simulink model "CAVE_MachE_Testing_testing_V2"  (R2024a)
settings: configuration reference "ConfigSetDesktopFixedStep" (kept outside this file)
PreLoadFcn:
  | VSS_BICYCLE=Simulink.Variant('Dual=0');
  | VSS_DUAL=Simulink.Variant('Dual=1');
  | Dual=1;
  | load('DriveCycle2.mat')
PostLoadFcn:
  | if any(exist('dsrtsu_mdlpostloadfcn', 'file') ~= 0), dsrtsu_mdlpostloadfcn('Execute', bdroot); end
InitFcn:
  | , if any(exist('rtifpga_mdlclblib', 'file') ~= 0), rtifpga_mdlclblib('Init', bdroot); end,
  | , if any(exist('dsmpb_private', 'file') ~= 0), dsmpb_private('dsmpb_mdlclblib', 'Init', bdroot); end,
  | load('DriveCycle2.mat')
model workspace (MAT data in the model file):
  Gas = 0.383333333333
undefined symbols (not defined in the file or in its folder): AccelCmd, ActTqLF_Nm_, ActTqLR_Nm_, ActTqRF_Nm_, ActTqRR_Nm_, BattChargeLimitMaxPwr, BattChargeLimitSocBpts, BattChargeLimitTbl, BattChrgCapcty, BattDischargeLimitSocBpts, BattDischargeLimitTbl, BattDischargeMaxPwr, BattNumCellsParallel, BattNumCellsSeries, BattOpenVoltCapBpts, BattOpenVoltTbl, BattResistSocBpts, BattResistTbl, BattResistTempBpts, BrakeMaxPrs, BrakeMaxTrq, ChassisDistCg2FrontAxle, ChassisDistCg2RearAxle, ChassisVehMass, CltchCmd, CoastDown, DecelCmd, DiffRatio, DiscIntNeverNeededParam, EnvGravCnst, EnvPrs, EnvTemp, FuelSpecificGrav, GearCmd, h, InitStates, lgSw, limitedMCT, MCT, MtrEffSpdBpts, MtrEffTbl, MtrEffTrqBpts, MtrPwrMax, MtrTrqMax, out_1, pMCT, RealSimPara, Ref_speed, Ref_time, SteeringCmd, SupvsryCtrlRegenBrkCutOffTbl, SupvsryCtrlRegenSpdBpts, TestScnrioCycleNum, US06, VEH
libraries: VSIGenLib x65, simulink x54, etargetslib x38, dsmpblib x24, vehdynlibtire x12, autolibshared x11, vehdynlibsuspension x7, vehdynlibtirecommon x7, autolibpowerinfoutils x6, autolibutils x5, autolibsharedcoupling x4, autolibmappedmotor x4
(part 9 of 17)

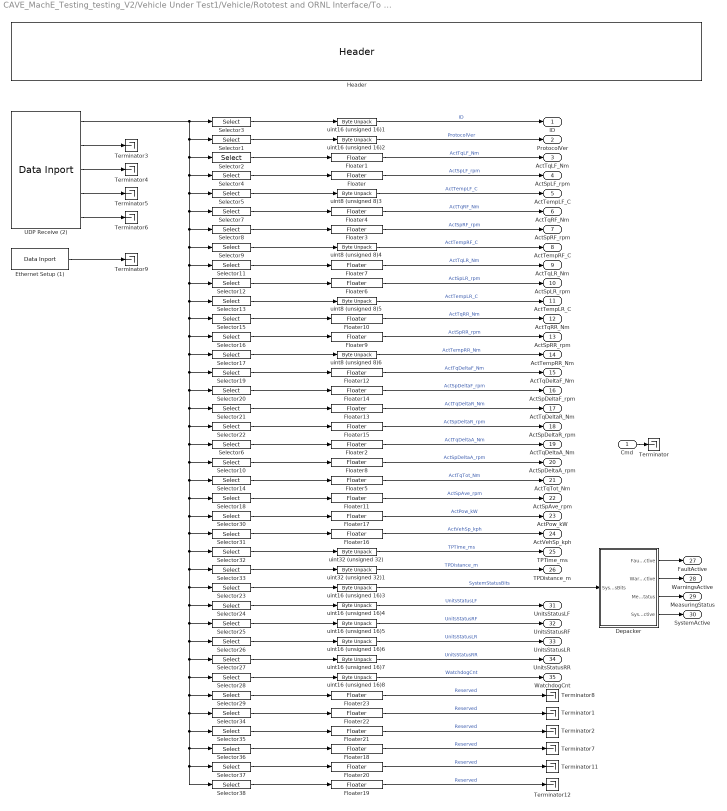
== system CAVE_MachE_Testing_testing_V2/Vehicle Under Test1/Vehicle/Rototest and ORNL Interface/To Rototest with Band-Aid/Logging/RotoTestEthRXLogging ==
  Cmd : Inport
  Depacker : Subsystem
  Ethernet Setup (1) : dsmpblib/Data Inport  Priority=10000
      settings: SourceProductName=dSPACE Model Interface Package for Simulink (MIPS)
  Floater{,1..23} (24 alike) : VSIGenLib/Floater  SystemSampleTime=-1  VariantActivationTime=update diagram  AllowFlexibleInterface=on  Latency=0  AutoFrameSizeCalculation=off
  Header : VSIGenLib/Header  not=''
  Selector1 : Selector  IndexMode=Zero-based  InputPortWidth=124  IndexOptions=Index vector (dialog)  Indices=[3 2]  OutputSizes=1
  Selector10 : Selector  IndexMode=Zero-based  InputPortWidth=124  IndexOptions=Index vector (dialog)  Indices=[63 62 61 60]  OutputSizes=1
  Selector11 : Selector  IndexMode=Zero-based  InputPortWidth=124  IndexOptions=Index vector (dialog)  Indices=[25 24 23 22]  OutputSizes=1
  Selector12 : Selector  IndexMode=Zero-based  InputPortWidth=124  IndexOptions=Index vector (dialog)  Indices=[29 28 27 26]  OutputSizes=1
  Selector13 : Selector  IndexMode=Zero-based  InputPortWidth=124  IndexOptions=Index vector (dialog)  Indices=[30]  OutputSizes=1
  Selector14 : Selector  IndexMode=Zero-based  InputPortWidth=124  IndexOptions=Index vector (dialog)  Indices=[67 66 65 64]  OutputSizes=1
  Selector15 : Selector  IndexMode=Zero-based  InputPortWidth=124  IndexOptions=Index vector (dialog)  Indices=[34 33 32 31]  OutputSizes=1
  Selector16 : Selector  IndexMode=Zero-based  InputPortWidth=124  IndexOptions=Index vector (dialog)  Indices=[38 37 36 35]  OutputSizes=1
  Selector17 : Selector  IndexMode=Zero-based  InputPortWidth=124  IndexOptions=Index vector (dialog)  Indices=[39]  OutputSizes=1
  Selector18 : Selector  IndexMode=Zero-based  InputPortWidth=124  IndexOptions=Index vector (dialog)  Indices=[71 70 69 68]  OutputSizes=1
  Selector19 : Selector  IndexMode=Zero-based  InputPortWidth=124  IndexOptions=Index vector (dialog)  Indices=[43 42 41 40]  OutputSizes=1
  Selector2 : Selector  IndexMode=Zero-based  InputPortWidth=124  IndexOptions=Index vector (dialog)  Indices=[7 6 5 4]  OutputSizes=1
  Selector20 : Selector  IndexMode=Zero-based  InputPortWidth=124  IndexOptions=Index vector (dialog)  Indices=[47 46 45 44]  OutputSizes=1
  Selector21 : Selector  IndexMode=Zero-based  InputPortWidth=124  IndexOptions=Index vector (dialog)  Indices=[51 50 49 48]  OutputSizes=1
  Selector22 : Selector  IndexMode=Zero-based  InputPortWidth=124  IndexOptions=Index vector (dialog)  Indices=[55 54 53 52]  OutputSizes=1
  Selector23 : Selector  IndexMode=Zero-based  InputPortWidth=124  IndexOptions=Index vector (dialog)  Indices=[89 88]  OutputSizes=1
  Selector24 : Selector  IndexMode=Zero-based  InputPortWidth=124  IndexOptions=Index vector (dialog)  Indices=[91 90]  OutputSizes=1
  Selector25 : Selector  IndexMode=Zero-based  InputPortWidth=124  IndexOptions=Index vector (dialog)  Indices=[93 92]  OutputSizes=1
  Selector26 : Selector  IndexMode=Zero-based  InputPortWidth=124  IndexOptions=Index vector (dialog)  Indices=[95 94]  OutputSizes=1
  Selector27 : Selector  IndexMode=Zero-based  InputPortWidth=124  IndexOptions=Index vector (dialog)  Indices=[97 96]  OutputSizes=1
  Selector28 : Selector  IndexMode=Zero-based  InputPortWidth=124  IndexOptions=Index vector (dialog)  Indices=[99 98]  OutputSizes=1
  Selector29 : Selector  IndexMode=Zero-based  InputPortWidth=124  IndexOptions=Index vector (dialog)  Indices=[103 102 101 100]  OutputSizes=1
  Selector3 : Selector  IndexMode=Zero-based  InputPortWidth=124  IndexOptions=Index vector (dialog)  Indices=[1 0]  OutputSizes=1
  Selector30 : Selector  IndexMode=Zero-based  InputPortWidth=124  IndexOptions=Index vector (dialog)  Indices=[67 66 65 64]  OutputSizes=1
  Selector31 : Selector  IndexMode=Zero-based  InputPortWidth=124  IndexOptions=Index vector (dialog)  Indices=[71 70 69 68]  OutputSizes=1
  Selector32 : Selector  IndexMode=Zero-based  InputPortWidth=124  IndexOptions=Index vector (dialog)  Indices=[83 82 81 80]  OutputSizes=1
  Selector33 : Selector  IndexMode=Zero-based  InputPortWidth=124  IndexOptions=Index vector (dialog)  Indices=[87 86 85 84]  OutputSizes=1
  Selector34 : Selector  IndexMode=Zero-based  InputPortWidth=124  IndexOptions=Index vector (dialog)  Indices=[107 106 105 104]  OutputSizes=1
  Selector35 : Selector  IndexMode=Zero-based  InputPortWidth=124  IndexOptions=Index vector (dialog)  Indices=[111 110 109 108]  OutputSizes=1
  Selector36 : Selector  IndexMode=Zero-based  InputPortWidth=124  IndexOptions=Index vector (dialog)  Indices=[115 114 113 112]  OutputSizes=1
  Selector37 : Selector  IndexMode=Zero-based  InputPortWidth=124  IndexOptions=Index vector (dialog)  Indices=[119 118 117 116]  OutputSizes=1
  Selector38 : Selector  IndexMode=Zero-based  InputPortWidth=124  IndexOptions=Index vector (dialog)  Indices=[123 122 121 120]  OutputSizes=1
  Selector4 : Selector  IndexMode=Zero-based  InputPortWidth=124  IndexOptions=Index vector (dialog)  Indices=[11 10 9 8]  OutputSizes=1
  Selector5 : Selector  IndexMode=Zero-based  InputPortWidth=124  IndexOptions=Index vector (dialog)  Indices=[12]  OutputSizes=1
  Selector6 : Selector  IndexMode=Zero-based  InputPortWidth=124  IndexOptions=Index vector (dialog)  Indices=[59 58 57 56]  OutputSizes=1
  Selector7 : Selector  IndexMode=Zero-based  InputPortWidth=124  IndexOptions=Index vector (dialog)  Indices=[16 15 14 13]  OutputSizes=1
  Selector8 : Selector  IndexMode=Zero-based  InputPortWidth=124  IndexOptions=Index vector (dialog)  Indices=[20 19 18 17]  OutputSizes=1
  Selector9 : Selector  IndexMode=Zero-based  InputPortWidth=124  IndexOptions=Index vector (dialog)  Indices=[21]  OutputSizes=1
  Terminator{,1..9,11..12} (12 alike) : Terminator
  UDP Receive (2) : dsmpblib/Data Inport  Priority=10000
      settings: SourceProductName=dSPACE Model Interface Package for Simulink (MIPS)
  uint16 (unsigned 16){1..8} (8 alike) : etargetslib/Byte Unpack  dimensions={[1]}  datatypes={'uint16'}  byteAlign=1
  uint32 (unsigned 32) : etargetslib/Byte Unpack  dimensions={[1]}  datatypes={'uint32'}  byteAlign=1
  uint32 (unsigned 32)1 : etargetslib/Byte Unpack  dimensions={[1]}  datatypes={'uint32'}  byteAlign=1
  uint8 (unsigned 8){3..6} (4 alike) : etargetslib/Byte Unpack  dimensions={[1]}  datatypes={'uint8'}  byteAlign=1
  ID : Outport
  ProtocolVer : Outport  Port=2
  ActTqLF_Nm : Outport  Port=3
  ActSpLF_rpm : Outport  Port=4
  ActTempLF_C : Outport  Port=5
  ActTqRF_Nm : Outport  Port=6
  ActSpRF_rpm : Outport  Port=7
  ActTempRF_C : Outport  Port=8
  ActTqLR_Nm : Outport  Port=9
  ActSpLR_rpm : Outport  Port=10
  ActTempLR_C : Outport  Port=11
  ActTqRR_Nm : Outport  Port=12
  ActSpRR_rpm : Outport  Port=13
  ActTempRR_Nm : Outport  Port=14
  ActTqDeltaF_Nm : Outport  Port=15
  ActSpDeltaF_rpm : Outport  Port=16
  ActTqDeltaR_Nm : Outport  Port=17
  ActSpDeltaR_rpm : Outport  Port=18
  ActTqDeltaA_Nm : Outport  Port=19
  ActSpDeltaA_rpm : Outport  Port=20
  ActTqTot_Nm : Outport  Port=21
  ActSpAve_rpm : Outport  Port=22
  ActPow_kW : Outport  Port=23
  ActVehSp_kph : Outport  Port=24
  TPTime_ms : Outport  Port=25
  TPDistance_m : Outport  Port=26
  FaultActive : Outport  Port=27
  WarningsActive : Outport  Port=28
  MeasuringStatus : Outport  Port=29
  SystemActive : Outport  Port=30
  UnitsStatusLF : Outport  Port=31
  UnitsStatusRF : Outport  Port=32
  UnitsStatusLR : Outport  Port=33
  UnitsStatusRR : Outport  Port=34
  WatchdogCnt : Outport  Port=35
  wires:
  Cmd/1 -> Terminator/1
  Floater23/1 -> Terminator8/1  "Reserved"
  Floater22/1 -> Terminator1/1  "Reserved"
  Floater21/1 -> Terminator2/1  "Reserved"
  Floater20/1 -> Terminator11/1  "Reserved"
  Floater19/1 -> Terminator12/1  "Reserved"
  Floater18/1 -> Terminator7/1  "Reserved"
  Selector38/1 -> Floater19/1
  UDP Receive (2)/1 -> Selector7/1, Selector8/1, Selector9/1, Selector11/1, Selector12/1, Selector13/1, Selector15/1, Selector16/1, Selector17/1, Selector19/1, Selector20/1, Selector21/1, Selector22/1, Selector6/1, Selector10/1, Selector14/1, Selector18/1, Selector30/1, Selector31/1, Selector32/1, Selector33/1, Selector23/1, Selector25/1, Selector26/1, Selector27/1, Selector29/1, Selector34/1, Selector35/1, Selector36/1, Selector37/1, Selector38/1, Selector28/1, Selector24/1, Selector5/1, Selector4/1, Selector2/1, Selector1/1, Selector3/1
  Selector37/1 -> Floater20/1
  Selector36/1 -> Floater18/1
  Selector35/1 -> Floater21/1
  Selector34/1 -> Floater22/1
  Selector32/1 -> uint32 (unsigned 32)/1
  Selector33/1 -> uint32 (unsigned 32)1/1
  uint32 (unsigned 32)1/1 -> TPDistance_m/1  "TPDistance_m"
  uint32 (unsigned 32)/1 -> TPTime_ms/1  "TPTime_ms"
  Floater16/1 -> ActVehSp_kph/1  "ActVehSp_kph"
  Selector31/1 -> Floater16/1
  Floater17/1 -> ActPow_kW/1  "ActPow_kW"
  Selector30/1 -> Floater17/1
  Selector6/1 -> Floater2/1
  Selector14/1 -> Floater5/1
  Selector10/1 -> Floater8/1
  Floater5/1 -> ActTqTot_Nm/1  "ActTqTot_Nm"
  Selector18/1 -> Floater11/1
  Floater2/1 -> ActTqDeltaA_Nm/1  "ActTqDeltaA_Nm"
  Floater8/1 -> ActSpDeltaA_rpm/1  "ActSpDeltaA_rpm"
  Floater11/1 -> ActSpAve_rpm/1  "ActSpAve_rpm"
  Ethernet Setup (1)/1 -> Terminator9/1
  Depacker/4(SystemActive) -> SystemActive/1
  Depacker/1(FaultActive) -> FaultActive/1
  Depacker/2(WarningsActive) -> WarningsActive/1
  Depacker/3(MeasuringStatus) -> MeasuringStatus/1
  uint8 (unsigned 8)4/1 -> ActTempRF_C/1  "ActTempRF_C"
  Floater/1 -> ActSpLF_rpm/1  "ActSpLF_rpm"
  uint16 (unsigned 16)1/1 -> ID/1  "ID"
  Floater15/1 -> ActSpDeltaR_rpm/1  "ActSpDeltaR_rpm"
  uint16 (unsigned 16)8/1 -> WatchdogCnt/1  "WatchdogCnt"
  Floater14/1 -> ActSpDeltaF_rpm/1  "ActSpDeltaF_rpm"
  uint16 (unsigned 16)5/1 -> UnitsStatusRF/1  "UnitsStatusRF"
  Floater9/1 -> ActSpRR_rpm/1  "ActSpRR_rpm"
  Floater1/1 -> ActTqLF_Nm/1  "ActTqLF_Nm"
  uint8 (unsigned 8)3/1 -> ActTempLF_C/1  "ActTempLF_C"
  Floater12/1 -> ActTqDeltaF_Nm/1  "ActTqDeltaF_Nm"
  Floater7/1 -> ActTqLR_Nm/1  "ActTqLR_Nm"
  uint16 (unsigned 16)2/1 -> ProtocolVer/1  "ProtocolVer"
  Selector24/1 -> uint16 (unsigned 16)4/1
  Selector7/1 -> Floater4/1
  Selector8/1 -> Floater3/1
  uint16 (unsigned 16)7/1 -> UnitsStatusRR/1  "UnitsStatusRR"
  Selector22/1 -> Floater15/1
  Selector12/1 -> Floater6/1
  Selector23/1 -> uint16 (unsigned 16)3/1
  uint16 (unsigned 16)6/1 -> UnitsStatusLR/1  "UnitsStatusLR"
  Selector17/1 -> uint8 (unsigned 8)6/1
  UDP Receive (2)/3 -> Terminator4/1
  uint16 (unsigned 16)4/1 -> UnitsStatusLF/1  "UnitsStatusLF"
  Selector27/1 -> uint16 (unsigned 16)7/1
  Floater13/1 -> ActTqDeltaR_Nm/1  "ActTqDeltaR_Nm"
  Selector2/1 -> Floater1/1
  Selector13/1 -> uint8 (unsigned 8)5/1
  Selector26/1 -> uint16 (unsigned 16)6/1
  uint16 (unsigned 16)3/1 -> Depacker/1(SysStsBits)  "SystemStatusBits"
  Floater3/1 -> ActSpRF_rpm/1  "ActSpRF_rpm"
  UDP Receive (2)/2 -> Terminator3/1
  Selector25/1 -> uint16 (unsigned 16)5/1
  Floater4/1 -> ActTqRF_Nm/1  "ActTqRF_Nm"
  Selector29/1 -> Floater23/1
  uint8 (unsigned 8)6/1 -> ActTempRR_Nm/1  "ActTempRR_Nm"
  Floater6/1 -> ActSpLR_rpm/1  "ActSpLR_rpm"
  Selector20/1 -> Floater14/1
  Selector9/1 -> uint8 (unsigned 8)4/1
  Selector5/1 -> uint8 (unsigned 8)3/1
  Selector15/1 -> Floater10/1
  Selector16/1 -> Floater9/1
  uint8 (unsigned 8)5/1 -> ActTempLR_C/1  "ActTempLR_C"
  Selector3/1 -> uint16 (unsigned 16)1/1
  UDP Receive (2)/4 -> Terminator5/1
  Selector28/1 -> uint16 (unsigned 16)8/1
  Selector21/1 -> Floater13/1
  Selector19/1 -> Floater12/1
  Selector1/1 -> uint16 (unsigned 16)2/1
  UDP Receive (2)/5 -> Terminator6/1
  Selector4/1 -> Floater/1
  Floater10/1 -> ActTqRR_Nm/1  "ActTqRR_Nm"
  Selector11/1 -> Floater7/1

== system CAVE_MachE_Testing_testing_V2/Vehicle Under Test1/Vehicle/Rototest and ORNL Interface/To Rototest with Band-Aid/RotoTestEthTx/Packer ==
  SpTqRR : Inport
  SpTqLR : Inport  Port=2
  SpTqRF : Inport  Port=3
  SpTqLF : Inport  Port=4
  SystemActive : Inport  Port=5
  Add : Sum  Inputs=++++++++  OutDataTypeStr=uint8
  Bit0 : Gain  OutDataTypeStr=uint8
  Bit1 : Gain  Gain=2  OutDataTypeStr=uint8
  Bit2 : Gain  Gain=4  OutDataTypeStr=Inherit: Inherit via back propagation
  Bit3 : Gain  Gain=8  OutDataTypeStr=uint8
  Bit4 : Gain  Gain=16  OutDataTypeStr=uint8
  Bit5 : Gain  Gain=32  OutDataTypeStr=uint8
  Bit6 : Gain  Gain=64  OutDataTypeStr=uint8
  Bit7 : Gain  Gain=128  OutDataTypeStr=uint8
  Ground11 : Ground
  Header : VSIGenLib/Header  not=''
  SystemCtrlBits : Outport
  wires:
  SpTqRF/1 -> Bit2/1
  SpTqLF/1 -> Bit1/1
  SpTqRR/1 -> Bit4/1
  SpTqLR/1 -> Bit3/1
  Add/1 -> SystemCtrlBits/1  "SystemCtrlBits"
  Bit0/1 -> Add/8  "SystemActive"
  Bit1/1 -> Add/7  "SpTqLF"
  Bit7/1 -> Add/1  "Reserved"
  SystemActive/1 -> Bit0/1
  Bit4/1 -> Add/4  "SpTqRR"
  Bit6/1 -> Add/2  "Reserved"
  Bit3/1 -> Add/5  "SpTqLR"
  Ground11/1 -> Bit7/1, Bit5/1, Bit6/1  "Reserved"
  Bit5/1 -> Add/3  "Reserved"
  Bit2/1 -> Add/6  "SpTqRF"

== system CAVE_MachE_Testing_testing_V2/Vehicle Under Test1/Vehicle/Vehicle Dynamics/Vehicle 14DOF/Subsystem1/Subsystem ==
  Cgxyzdot : Inport
  angles : Inport  Port=2
  Demux2 : Demux  Outputs=3
  Demux3 : Demux  Outputs=3
  Scope : Scope
  Terminator{,1..4} (5 alike) : Terminator
  VehSpd : Outport
  wires:
  Cgxyzdot/1 -> Demux2/1
  Demux3/2 -> Terminator3/1  "theta"
  Demux2/2 -> Scope/1, Terminator/1  "xdot"
  Demux3/1 -> Terminator2/1  "phi"
  Demux3/3 -> Terminator4/1  "psi"
  Demux2/3 -> Terminator1/1  "zdot"
  angles/1 -> Demux3/1
  Demux2/1 -> VehSpd/1  "xdot"

== system CAVE_MachE_Testing_testing_V2/Vehicle Under Test1/Vehicle/Vehicle Dynamics/Vehicle 14DOF/Subsystem4/Subsystem ==
  Cgxyzdot : Inport
  angles : Inport  Port=2
  Demux2 : Demux  Outputs=3
  Demux3 : Demux  Outputs=3
  Terminator{,1..4} (5 alike) : Terminator
  VehSpd : Outport
  wires:
  Demux2/1 -> VehSpd/1  "xdot"
  angles/1 -> Demux3/1
  Demux2/3 -> Terminator1/1  "zdot"
  Demux3/3 -> Terminator4/1  "psi"
  Demux3/1 -> Terminator2/1  "phi"
  Demux2/2 -> Terminator/1  "xdot"
  Demux3/2 -> Terminator3/1  "theta"
  Cgxyzdot/1 -> Demux2/1

== system CAVE_MachE_Testing_testing_V2/Vehicle Under Test1/Vehicle/Vehicle Dynamics/Vehicle 14DOF/Suspension/Double Wishbone Suspension ==
  Wheel : Inport
  Steering : Inport  Port=2
  Vehicle : Inport  Port=3
  Bus Creator1 : BusCreator  Inputs=5
  Bus Creator2 : BusCreator  Inputs=2
  Bus Creator3 : BusCreator  Inputs=2
  Bus Creator4 : BusCreator  Inputs=6
  Bus Selector : BusSelector  OutputSignals=z,Re,zdot,Fx,Fy,M
  Bus Selector1 : BusSelector  OutputSignals=P,V
  Independent Suspension – Double Wishbone : vehdynlibsuspension/Independent Suspension - Double Wishbone  ActiveDampEn=off  NumAxl=2  NumWhlsByAxl=[2 2]  StrgEnByAxl=[1 0]  AntiSwayEnByAxl=[1 0]  WhlNumVec="[1  2  1  2]"  AxleNumVec="[1  1  2  2]"  SuspTypesByAxle="[1  1]"  SuspImage=suspdw.png  IdealSuspEn=on  IdealSuspAxles="[1  2]"  Kz=Kz  F0z=F0z  Cz=Cz  Hmax=Hmax  f_act_susp_cz=[10000 10000;10000 10000]  f_act_susp_duty_bpt=[0 1]  f_act_susp_zdot_bpt=[-1 1]  Toe=0.  RollStrgSlp=0.  ToeStrgSlp=0.  Caster=0.  CasterHslp=0.  CasterStrgSlp=0.  Camber=0.  CamberHslp=0.  CamberStrgSlp=0.  StrgHgtSlp=0.1432  MappedSuspEn=off  MappedSuspAxles="[1  2]"  f_susp_axl_bp=[1 2]  f_susp_dz_bp=[-0.15 -0.14 -0.13 -0.12 -0.11 -0.10 -0.09 -0.08 -0.07 -0.06 -0.05 -0.04 -0.03 -0.02 -0.01 0.00 0.01 0.02 0.03 0.04 0.05 0.06 0.07 0.08 0.09 0.10 0.11 0.12 0.13 0.14 0.15]  f_susp_dzdot_bp=[-0.15 -0.14 -0.13 -0.12 -0.11 -0.10 -0.09 -0.08 -0.07 -0.06 -0.05 -0.04 -0.03 -0.02 -0.01 0.00 0.01 0.02 0.03 0.04 0.05 0.06 0.07 0.08 0.09 0.10 0.11 0.12 0.13 0.14 0.15]  f_susp_fmz=zeros(31,31,61,2,4)  f_susp_geom=zeros(31,61,2,3)  f_susp_strgdelta_bp=[-30,-29,-28,-27,-26,-25,-24,-23,-22,-21,-20,-19,-18,-17,-16,-15,-14,-13,-12,-11,-10,-9,-8,-7,-6,-5,-4,-3,-2,-1,0,1,2,3,4,5,6,7,8,9,10,11,12,13,14,15,16,17,18,19,20,21,22,23,24,25,26,27,28,29,30]  AntiSwayR=0.2  AntiSwayNtrlAng=0.5236  AntiSwayTrsK=8e2
  Selector1 : Selector  NumberOfDimensions=2  IndexOptions=Index vector (dialog),Select all  Indices=1,1  OutputSizes=1,1
  Selector2 : Selector  NumberOfDimensions=2  IndexOptions=Index vector (dialog),Select all  Indices=2,1  OutputSizes=1,1
  Steer Rate Adapter : Subsystem
  Steering Adapter : Subsystem
  Terminator : Terminator
  Vehicle Adapter : Subsystem
  Wheel  Adapter : Subsystem
  Suspension : Outport  VectorParamsAs1DForOutWhenUnconnected=off
  wires:
  Bus Selector/3 -> Independent Suspension – Double Wishbone/3  "<zdot>"
  Wheel  Adapter/1(WhlFx) -> Bus Creator4/1  "Fx"
  Bus Creator1/1 -> Bus Creator3/2  "Whl"
  Independent Suspension – Double Wishbone/6 -> Bus Creator1/4  "Ang"
  Wheel  Adapter/3(z) -> Bus Creator4/3
  Bus Selector/1 -> Independent Suspension – Double Wishbone/1  "<z>"
  Bus Selector/5 -> Independent Suspension – Double Wishbone/5  "<Fy>"
  Bus Selector/6 -> Independent Suspension – Double Wishbone/6  "<M>"
  Vehicle/1 -> Vehicle Adapter/1(Veh), Steer Rate Adapter/1(Veh)
  Wheel  Adapter/4(zdot) -> Bus Creator4/4
  Vehicle Adapter/1(VehSusp) -> Bus Selector1/1
  Independent Suspension – Double Wishbone/3 -> Bus Creator2/2  "M"
  Selector1/1 -> Bus Creator1/2  "xdot"
  Steering/1 -> Steering Adapter/1(Steer)
  Independent Suspension – Double Wishbone/4 -> Bus Creator1/1  "F"
  Bus Selector/4 -> Independent Suspension – Double Wishbone/4  "<Fx>"
  Wheel  Adapter/5(M) -> Bus Creator4/5  "M"
  Bus Selector/2 -> Independent Suspension – Double Wishbone/2  "<Re>"
  Independent Suspension – Double Wishbone/2 -> Bus Creator2/1  "F"
  Bus Selector1/2 -> Independent Suspension – Double Wishbone/8  "<V>"
  Selector2/1 -> Bus Creator1/3  "ydot"
  Independent Suspension – Double Wishbone/5 -> Selector1/1, Selector2/1  "V"
  Bus Creator2/1 -> Bus Creator3/1  "Veh"
  Bus Creator4/1 -> Bus Selector/1
  Steer Rate Adapter/1(AngVel) -> Bus Creator1/5  "AngVel"
  Wheel/1 -> Wheel  Adapter/1(Wheels)
  Wheel  Adapter/2(WhlFy) -> Bus Creator4/2  "Fy"
  Bus Selector1/1 -> Independent Suspension – Double Wishbone/7  "<P>"
  Wheel  Adapter/6(Re) -> Bus Creator4/6
  Independent Suspension – Double Wishbone/1 -> Terminator/1  "Susp"
  Steering Adapter/1(StrgAng) -> Independent Suspension – Double Wishbone/9
  Bus Creator3/1 -> Suspension/1

== system CAVE_MachE_Testing_testing_V2/Vehicle Under Test1/Vehicle/Vehicle Dynamics/Vehicle 14DOF/Suspension/Independent Mapped Front Suspension Mapped Solid Axle Rear Suspension ==
  Wheel : Inport
  Steering : Inport  Port=2
  Vehicle : Inport  Port=3
  Bus Creator1 : BusCreator  Inputs=5
  Bus Creator2 : BusCreator  Inputs=2
  Bus Creator3 : BusCreator  Inputs=2
  Bus Creator4 : BusCreator  Inputs=6
  Bus Selector : BusSelector  OutputSignals=z,Re,zdot,Fx,Fy,M
  Bus Selector1 : BusSelector  OutputSignals=P,V
  Independent Suspension - Mapped : vehdynlibsuspension/Independent Suspension - Mapped  NumAxl=1  NumWhlsByAxl=[2 2]  StrgEnByAxl=1  AntiSwayEnByAxl=1  WhlNumVec="[1  2  1  2]"  AxleNumVec="[1  1]"  SuspTypesByAxle=[2]  SuspImage=suspindmap.png  IdealSuspEn=off  IdealSuspAxles="[1  2]"  Kz=64370  F0z=9810  Cz=10000  Hmax=0.5  Toe=2  RollStrgSlp=-13  ToeStrgSlp=0.01  Caster=4  CasterHslp=-13  CasterStrgSlp=0.01  Camber=4  CamberHslp=-13  CamberStrgSlp=0.01  StrgHgtSlp=0.0025  MappedSuspEn=on  MappedSuspAxles=[1]  f_susp_axl_bp=[1 2]  f_susp_dz_bp=f_susp_dz_bp  f_susp_dzdot_bp=f_susp_dzdot_bp  f_susp_fmz=f_susp_fmz  f_susp_geom=f_susp_geom  f_susp_strgdelta_bp=f_susp_strgdelta_bp  NDFLookupOutType=1:4  NDGLookupOutType=1:3  AntiSwayR=0.2  AntiSwayNtrlAng=0.5236  AntiSwayTrsK=8e2
      link override For each track and axle combination calculate suspension forces and moments/Suspension/Suspension Angle Calculations: OverrideUsingVariant=MappedSteeringEnabled
      link override For each track and axle combination calculate suspension forces and moments/Suspension/Z axis suspension characteristic: OverrideUsingVariant=MappedSuspension
  Matrix Concatenate{,1..2,4..6} (6 alike) : Concatenate  Mode=Multidimensional array  ConcatenateDimension=2
  Selector1 : Selector  NumberOfDimensions=2  IndexOptions=Select all,Index vector (dialog)  Indices=[1 2],[3 4]  OutputSizes=1,1
  Selector10 : Selector  NumberOfDimensions=2  IndexOptions=Select all,Index vector (dialog)  Indices=[1 2],[1 2]  OutputSizes=1,1
  Selector11 : Selector  NumberOfDimensions=2  IndexOptions=Select all,Index vector (dialog)  Indices=[1 2],[1 2]  OutputSizes=1,1
  Selector12 : Selector  NumberOfDimensions=2  InputPortWidth=3  IndexOptions=Index vector (dialog),Select all  Indices=1,1  OutputSizes=1,1
  Selector13 : Selector  NumberOfDimensions=2  InputPortWidth=3  IndexOptions=Index vector (dialog),Select all  Indices=2,1  OutputSizes=1,1
  Selector14 : Selector  NumberOfDimensions=2  InputPortWidth=3  IndexOptions=Index vector (dialog),Select all  Indices=1,1  OutputSizes=1,1
  Selector15 : Selector  NumberOfDimensions=2  InputPortWidth=3  IndexOptions=Index vector (dialog),Select all  Indices=2,1  OutputSizes=1,1
  Selector{3,16,20..22} (5 alike) : Selector  IndexOptions=Index vector (dialog)  Indices=[3 4]  OutputSizes=1
  Selector17 : Selector  NumberOfDimensions=2  IndexOptions=Select all,Index vector (dialog)  Indices=[1 2],[3 4]  OutputSizes=1,1
  Selector18 : Selector  NumberOfDimensions=2  IndexOptions=Select all,Index vector (dialog)  Indices=[1 2],[3 4]  OutputSizes=1,1
  Selector{2,4..8} (6 alike) : Selector  IndexOptions=Index vector (dialog)  Indices=[1 2]  OutputSizes=1
  Selector9 : Selector  NumberOfDimensions=2  IndexOptions=Select all,Index vector (dialog)  Indices=[1 2],[1 2]  OutputSizes=1,1
  Solid Axle Suspension - Mapped : vehdynlibsuspension/Solid Axle Suspension - Mapped  NumAxl=1  NumWhlsByAxl=[2 2]  StrgEnByAxl=0  WhlNumVec="[1  2  1  2]"  AxleNumVec="[1  1]"  SuspTypesByAxle=[2]  SuspImage=suspsamap.png  AxlIxx=AxlIxx  AxlM=AxlM  TrackCoords=[0 0;VEH.TrackWidth*[-1 1]/2;0 0]  SuspCoords=[0 0;VEH.TrackWidth*[-1 1]/2;0 0]  KzWhlAxl=KzWhlAxl  F0zWhlAxl=F0zWhlAxl  CzWhlAxl=CzWhlAxl  IdealSuspEn=off  IdealSuspAxles="[1  2]"  Kz=64370  F0z=9810  Cz=10000  Hmax=0.5  Toe=2  RollStrgSlp=-13  ToeStrgSlp=0.01  Caster=4  CasterHslp=-13  CasterStrgSlp=0.01  Camber=4  CamberHslp=-13  CamberStrgSlp=0.01  StrgHgtSlp=0.0025  MappedSuspEn=on  MappedSuspAxles=[1]  f_susp_axl_bp=[1 2]  f_susp_dz_bp=f_susp_dz_bp  f_susp_dzdot_bp=f_susp_dzdot_bp  f_susp_fmz=f_susp_fmz  f_susp_geom=f_susp_geom  f_susp_strgdelta_bp=f_susp_strgdelta_bp  NDFLookupOutType=1:4  NDGLookupOutType=1:3
      link override For each track and axle combination calculate suspension forces and moments/Suspension/Suspension Angle Calculations: OverrideUsingVariant=MappedSteeringEnabled
      link override For each track and axle combination calculate suspension forces and moments/Suspension/Z axis suspension characteristic: OverrideUsingVariant=MappedSuspension
  Steer Rate Adapter : Subsystem
  Steering Adapter : Subsystem
  Terminator : Terminator
  Terminator1 : Terminator
  Vehicle Adapter : Subsystem
  Wheel  Adapter : Subsystem
  Suspension : Outport  VectorParamsAs1DForOutWhenUnconnected=off
  wires:
  Steer Rate Adapter/1(AngVel) -> Bus Creator1/5
  Bus Selector/2 -> Selector4/1, Selector20/1  "<Re>"
  Bus Creator3/1 -> Suspension/1
  Bus Creator1/1 -> Bus Creator3/2  "Whl"
  Bus Selector/5 -> Selector16/1, Selector8/1  "<Fy>"
  Bus Selector/1 -> Selector5/1, Selector3/1  "<z>"
  Solid Axle Suspension - Mapped/6 -> Matrix Concatenate2/2
  Bus Selector1/1 -> Selector1/1, Selector10/1  "<P>"
  Matrix Concatenate6/1 -> Bus Creator2/1  "F"
  Wheel  Adapter/6(Re) -> Bus Creator4/6
  Selector11/1 -> Independent Suspension - Mapped/8
  Wheel  Adapter/1(WhlFx) -> Bus Creator4/1  "Fx"
  Bus Selector/6 -> Selector17/1, Selector9/1  "<M>"
  Selector6/1 -> Independent Suspension - Mapped/3
  Steering Adapter/1(StrgAng) -> Selector2/1
  Vehicle Adapter/1(VehSusp) -> Bus Selector1/1
  Bus Selector1/2 -> Selector18/1, Selector11/1  "<V>"
  Selector3/1 -> Solid Axle Suspension - Mapped/1
  Selector15/1 -> Matrix Concatenate/2
  Matrix Concatenate1/1 -> Bus Creator1/2  "xdot"
  Steering/1 -> Steering Adapter/1(Steer)
  Matrix Concatenate/1 -> Bus Creator1/3  "ydot"
  Wheel  Adapter/5(M) -> Bus Creator4/5
  Selector2/1 -> Independent Suspension - Mapped/9
  Selector17/1 -> Solid Axle Suspension - Mapped/6
  Bus Creator4/1 -> Bus Selector/1
  Wheel  Adapter/2(WhlFy) -> Bus Creator4/2  "Fy"
  Matrix Concatenate2/1 -> Bus Creator1/4  "Ang"
  Independent Suspension - Mapped/5 -> Selector13/1, Selector12/1
  Bus Selector/4 -> Selector21/1, Selector7/1  "<Fx>"
  Bus Creator2/1 -> Bus Creator3/1  "Veh"
  Independent Suspension - Mapped/1 -> Terminator/1  "FSusp"
  Selector20/1 -> Solid Axle Suspension - Mapped/2
  Independent Suspension - Mapped/6 -> Matrix Concatenate2/1
  Independent Suspension - Mapped/2 -> Matrix Concatenate6/1
  Selector8/1 -> Independent Suspension - Mapped/5
  Independent Suspension - Mapped/3 -> Matrix Concatenate5/1
  Selector5/1 -> Independent Suspension - Mapped/1
  Wheel/1 -> Wheel  Adapter/1(Wheels)
  Solid Axle Suspension - Mapped/2 -> Matrix Concatenate6/2
  Wheel  Adapter/3(z) -> Bus Creator4/3
  Selector9/1 -> Independent Suspension - Mapped/6
  Selector10/1 -> Independent Suspension - Mapped/7
  Selector4/1 -> Independent Suspension - Mapped/2
  Independent Suspension - Mapped/4 -> Matrix Concatenate4/1
  Matrix Concatenate5/1 -> Bus Creator2/2  "M"
  Selector16/1 -> Solid Axle Suspension - Mapped/5
  Matrix Concatenate4/1 -> Bus Creator1/1  "F"
  Selector1/1 -> Solid Axle Suspension - Mapped/7
  Solid Axle Suspension - Mapped/3 -> Matrix Concatenate5/2
  Wheel  Adapter/4(zdot) -> Bus Creator4/4
  Vehicle/1 -> Vehicle Adapter/1(Veh), Steer Rate Adapter/1(Veh)
  Selector21/1 -> Solid Axle Suspension - Mapped/4
  Selector14/1 -> Matrix Concatenate1/2
  Selector13/1 -> Matrix Concatenate/1
  Selector18/1 -> Solid Axle Suspension - Mapped/8
  Selector7/1 -> Independent Suspension - Mapped/4
  Selector12/1 -> Matrix Concatenate1/1
  Solid Axle Suspension - Mapped/1 -> Terminator1/1  "Susp"
  Solid Axle Suspension - Mapped/4 -> Matrix Concatenate4/2
  Bus Selector/3 -> Selector6/1, Selector22/1  "<zdot>"
  Selector22/1 -> Solid Axle Suspension - Mapped/3
  Solid Axle Suspension - Mapped/5 -> Selector14/1, Selector15/1

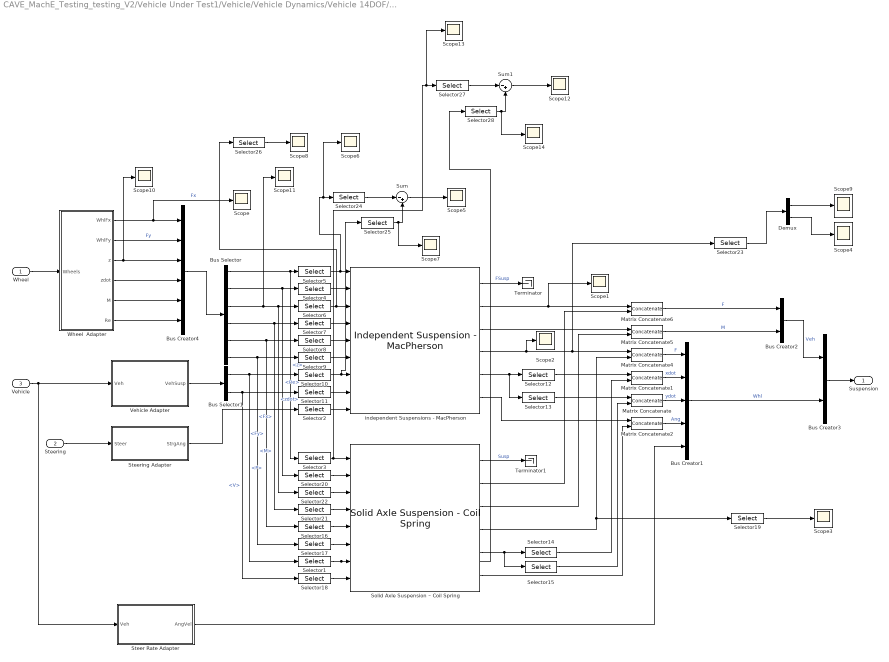
== system CAVE_MachE_Testing_testing_V2/Vehicle Under Test1/Vehicle/Vehicle Dynamics/Vehicle 14DOF/Suspension/MacPherson Front Suspension Solid Axle Rear Suspension ==
  Wheel : Inport
  Steering : Inport  Port=2
  Vehicle : Inport  Port=3
  Bus Creator1 : BusCreator  Inputs=5
  Bus Creator2 : BusCreator  Inputs=2
  Bus Creator3 : BusCreator  Inputs=2
  Bus Creator4 : BusCreator  Inputs=6
  Bus Selector : BusSelector  OutputSignals=z,Re,zdot,Fx,Fy,M
  Bus Selector1 : BusSelector  OutputSignals=P,V
  Demux : Demux  Outputs=2
  Matrix Concatenate{,1..2,4..6} (6 alike) : Concatenate  Mode=Multidimensional array  ConcatenateDimension=2
  Scope{,1..14} (15 alike) : Scope
  Selector1 : Selector  NumberOfDimensions=2  IndexOptions=Select all,Index vector (dialog)  Indices=[1 2],[3 4]  OutputSizes=1,1
  Selector10 : Selector  NumberOfDimensions=2  IndexOptions=Select all,Index vector (dialog)  Indices=[1 2],[1 2]  OutputSizes=1,1
  Selector11 : Selector  NumberOfDimensions=2  IndexOptions=Select all,Index vector (dialog)  Indices=[1 2],[1 2]  OutputSizes=1,1
  Selector12 : Selector  NumberOfDimensions=2  InputPortWidth=3  IndexOptions=Index vector (dialog),Select all  Indices=1,1  OutputSizes=1,1
  Selector13 : Selector  NumberOfDimensions=2  InputPortWidth=3  IndexOptions=Index vector (dialog),Select all  Indices=2,1  OutputSizes=1,1
  Selector14 : Selector  NumberOfDimensions=2  InputPortWidth=3  IndexOptions=Index vector (dialog),Select all  Indices=1,1  OutputSizes=1,1
  Selector15 : Selector  NumberOfDimensions=2  InputPortWidth=3  IndexOptions=Index vector (dialog),Select all  Indices=2,1  OutputSizes=1,1
  Selector{3,16,20..22} (5 alike) : Selector  IndexOptions=Index vector (dialog)  Indices=[3 4]  OutputSizes=1
  Selector17 : Selector  NumberOfDimensions=2  IndexOptions=Select all,Index vector (dialog)  Indices=[1 2],[3 4]  OutputSizes=1,1
  Selector18 : Selector  NumberOfDimensions=2  IndexOptions=Select all,Index vector (dialog)  Indices=[1 2],[3 4]  OutputSizes=1,1
  Selector19 : Selector  NumberOfDimensions=2  InputPortWidth=3  IndexOptions=Index vector (dialog),Select all  Indices=3,1  OutputSizes=1,1
  Selector{2,4..8} (6 alike) : Selector  IndexOptions=Index vector (dialog)  Indices=[1 2]  OutputSizes=1
  Selector23 : Selector  NumberOfDimensions=2  InputPortWidth=3  IndexOptions=Index vector (dialog),Select all  Indices=3,1  OutputSizes=1,1
  Selector24 : Selector  IndexOptions=Index vector (dialog)  Indices=[1]  OutputSizes=1
  Selector25 : Selector  NumberOfDimensions=2  IndexOptions=Index vector (dialog),Index vector (dialog)  Indices=[3],[1]  OutputSizes=1,1
  Selector26 : Selector  IndexOptions=Index vector (dialog)  Indices=[1]  OutputSizes=1
  Selector27 : Selector  IndexOptions=Index vector (dialog)  Indices=[1]  OutputSizes=1
  Selector28 : Selector  NumberOfDimensions=2  IndexOptions=Index vector (dialog),Index vector (dialog)  Indices=[3],[1]  OutputSizes=1,1
  Selector9 : Selector  NumberOfDimensions=2  IndexOptions=Select all,Index vector (dialog)  Indices=[1 2],[1 2]  OutputSizes=1,1
  Solid Axle Suspension – Coil Spring : vehdynlibsuspension/Solid Axle Suspension - Coil Spring  NumAxl=1  NumWhlsByAxl=2  StrgEnByAxl=0  WhlNumVec="[1  2]"  AxleNumVec="[1  1]"  SuspTypesByAxle=[1]  SuspImage=suspsacoil.png  AxlIxx=62  AxlM=160  TrackCoords=[0 0;1.9*[-1 1]/2;0 0]  SuspCoords=[0 0;1.9*[-1 1]/2;0 0]  KzWhlAxl=138031  F0zWhlAxl=5003*1  CzWhlAxl=11490  IdealSuspEn=on  IdealSuspAxles=[1]  Kz=52451*1  F0z=5003*1  Cz=5565*1  Hmax=0.32  Toe=0.  RollStrgSlp=0.  ToeStrgSlp=0  Caster=0.  CasterHslp=0.  CasterStrgSlp=0.01  Camber=0.  CamberHslp=0.  CamberStrgSlp=0.01  StrgHgtSlp=0.1432  MappedSuspEn=off  MappedSuspAxles="[1  2]"  f_susp_axl_bp=[1 2]  f_susp_dz_bp=[-0.15 -0.14 -0.13 -0.12 -0.11 -0.10 -0.09 -0.08 -0.07 -0.06 -0.05 -0.04 -0.03 -0.02 -0.01 0.00 0.01 0.02 0.03 0.04 0.05 0.06 0.07 0.08 0.09 0.10 0.11 0.12 0.13 0.14 0.15]  f_susp_dzdot_bp=[-0.15 -0.14 -0.13 -0.12 -0.11 -0.10 -0.09 -0.08 -0.07 -0.06 -0.05 -0.04 -0.03 -0.02 -0.01 0.00 0.01 0.02 0.03 0.04 0.05 0.06 0.07 0.08 0.09 0.10 0.11 0.12 0.13 0.14 0.15]  f_susp_fmz=zeros(31,31,61,2,4)  f_susp_geom=zeros(31,61,2,3)  f_susp_strgdelta_bp=[-30,-29,-28,-27,-26,-25,-24,-23,-22,-21,-20,-19,-18,-17,-16,-15,-14,-13,-12,-11,-10,-9,-8,-7,-6,-5,-4,-3,-2,-1,0,1,2,3,4,5,6,7,8,9,10,11,12,13,14,15,16,17,18,19,20,21,22,23,24,25,26,27,28,29,30]
  Steer Rate Adapter : Subsystem
  Steering Adapter : Subsystem
  Sum : Sum  Inputs=|-+
  Sum1 : Sum  Inputs=|-+
  Terminator : Terminator
  Terminator1 : Terminator
  Vehicle Adapter : Subsystem
  Wheel  Adapter : Subsystem
  independent Suspensions - MacPherson : vehdynlibsuspension/Independent Suspension - MacPherson  ActiveDampEn=off  NumAxl=1  NumWhlsByAxl=2  StrgEnByAxl=1  AntiSwayEnByAxl=1  WhlNumVec="[1  2]"  AxleNumVec="[1  1]"  SuspTypesByAxle=[1]  SuspImage=suspmacp.png  IdealSuspEn=on  IdealSuspAxles=[1]  Kz=52451*1  F0z=5003*1  Cz=5565*1  Hmax=0.32  f_act_susp_cz=[10000 10000;10000 10000]  f_act_susp_duty_bpt=[0 1]  f_act_susp_zdot_bpt=[-1 1]  Toe=0.  RollStrgSlp=0.  ToeStrgSlp=0.  Caster=0.  CasterHslp=0.  CasterStrgSlp=0.  Camber=0.  CamberHslp=0.  CamberStrgSlp=0.  StrgHgtSlp=0.1432  MappedSuspEn=off  MappedSuspAxles="[1  2]"  f_susp_axl_bp=[1 2]  f_susp_dz_bp=[-0.15 -0.14 -0.13 -0.12 -0.11 -0.10 -0.09 -0.08 -0.07 -0.06 -0.05 -0.04 -0.03 -0.02 -0.01 0.00 0.01 0.02 0.03 0.04 0.05 0.06 0.07 0.08 0.09 0.10 0.11 0.12 0.13 0.14 0.15]  f_susp_dzdot_bp=[-0.15 -0.14 -0.13 -0.12 -0.11 -0.10 -0.09 -0.08 -0.07 -0.06 -0.05 -0.04 -0.03 -0.02 -0.01 0.00 0.01 0.02 0.03 0.04 0.05 0.06 0.07 0.08 0.09 0.10 0.11 0.12 0.13 0.14 0.15]  f_susp_fmz=zeros(31,31,61,2,4)  f_susp_geom=zeros(31,61,2,3)  f_susp_strgdelta_bp=[-30,-29,-28,-27,-26,-25,-24,-23,-22,-21,-20,-19,-18,-17,-16,-15,-14,-13,-12,-11,-10,-9,-8,-7,-6,-5,-4,-3,-2,-1,0,1,2,3,4,5,6,7,8,9,10,11,12,13,14,15,16,17,18,19,20,21,22,23,24,25,26,27,28,29,30]  AntiSwayR=0.2  AntiSwayNtrlAng=0.5236  AntiSwayTrsK=8e+02
  Suspension : Outport  VectorParamsAs1DForOutWhenUnconnected=off
  wires:
  Steer Rate Adapter/1(AngVel) -> Bus Creator1/5
  Solid Axle Suspension – Coil Spring/5 -> Selector14/1, Selector15/1
  Solid Axle Suspension – Coil Spring/1 -> Terminator1/1  "Susp"
  Bus Selector/3 -> Scope11/1, Selector6/1, Selector22/1  "<zdot>"
  Selector22/1 -> Solid Axle Suspension – Coil Spring/3
  Vehicle/1 -> Vehicle Adapter/1(Veh), Steer Rate Adapter/1(Veh)
  Solid Axle Suspension – Coil Spring/3 -> Matrix Concatenate5/2
  Selector21/1 -> Solid Axle Suspension – Coil Spring/4
  Wheel  Adapter/6(Re) -> Bus Creator4/6
  Selector20/1 -> Solid Axle Suspension – Coil Spring/2
  Selector18/1 -> Solid Axle Suspension – Coil Spring/8
  Selector17/1 -> Solid Axle Suspension – Coil Spring/6
  Selector16/1 -> Solid Axle Suspension – Coil Spring/5
  Solid Axle Suspension – Coil Spring/2 -> Matrix Concatenate6/2
  Matrix Concatenate6/1 -> Bus Creator2/1  "F"
  Matrix Concatenate5/1 -> Bus Creator2/2  "M"
  Solid Axle Suspension – Coil Spring/4 -> Selector19/1, Matrix Concatenate4/2
  Matrix Concatenate4/1 -> Bus Creator1/1  "F"
  Solid Axle Suspension – Coil Spring/6 -> Matrix Concatenate2/2
  Matrix Concatenate2/1 -> Bus Creator1/4  "Ang"
  Selector14/1 -> Matrix Concatenate1/2
  Matrix Concatenate1/1 -> Bus Creator1/2  "xdot"
  Selector15/1 -> Matrix Concatenate/2
  Selector13/1 -> Matrix Concatenate/1
  Selector11/1 -> independent Suspensions - MacPherson/8
  Selector10/1 -> Selector25/1, independent Suspensions - MacPherson/7
  Selector9/1 -> independent Suspensions - MacPherson/6
  Selector8/1 -> independent Suspensions - MacPherson/5
  Selector7/1 -> independent Suspensions - MacPherson/4
  Selector6/1 -> Selector26/1, independent Suspensions - MacPherson/3
  Selector5/1 -> Scope6/1, Selector24/1, independent Suspensions - MacPherson/1
  Selector4/1 -> independent Suspensions - MacPherson/2
  Selector2/1 -> independent Suspensions - MacPherson/9
  Bus Selector/2 -> Selector4/1, Selector20/1  "<Re>"
  Wheel  Adapter/5(M) -> Bus Creator4/5
  Wheel  Adapter/4(zdot) -> Bus Creator4/4
  Wheel  Adapter/3(z) -> Scope10/1, Bus Creator4/3
  Wheel/1 -> Wheel  Adapter/1(Wheels)
  Wheel  Adapter/1(WhlFx) -> Bus Creator4/1, Scope/1  "Fx"
  Wheel  Adapter/2(WhlFy) -> Bus Creator4/2  "Fy"
  Bus Creator4/1 -> Bus Selector/1
  Steering Adapter/1(StrgAng) -> Selector2/1
  Bus Creator2/1 -> Bus Creator3/1  "Veh"
  independent Suspensions - MacPherson/3 -> Matrix Concatenate5/1
  independent Suspensions - MacPherson/2 -> Matrix Concatenate6/1, Scope1/1
  Vehicle Adapter/1(VehSusp) -> Bus Selector1/1
  Bus Selector/4 -> Selector21/1, Selector7/1  "<Fx>"
  independent Suspensions - MacPherson/1 -> Terminator/1  "FSusp"
  independent Suspensions - MacPherson/4 -> Selector23/1, Matrix Concatenate4/1, Scope2/1
  Selector12/1 -> Matrix Concatenate1/1
  independent Suspensions - MacPherson/6 -> Matrix Concatenate2/1
  independent Suspensions - MacPherson/5 -> Selector13/1, Selector12/1
  Matrix Concatenate/1 -> Bus Creator1/3  "ydot"
  Bus Selector1/1 -> Selector1/1, Selector10/1  "<P>"
  Steering/1 -> Steering Adapter/1(Steer)
  Bus Selector/1 -> Selector5/1, Selector3/1  "<z>"
  Bus Selector/5 -> Selector16/1, Selector8/1  "<Fy>"
  Bus Selector/6 -> Selector17/1, Selector9/1  "<M>"
  Bus Selector1/2 -> Selector18/1, Selector11/1  "<V>"
  Bus Creator1/1 -> Bus Creator3/2  "Whl"
  Bus Creator3/1 -> Suspension/1
  Selector19/1 -> Scope3/1
  Selector23/1 -> Demux/1
  Selector24/1 -> Sum/1
  Selector25/1 -> Scope7/1, Sum/2
  Sum/1 -> Scope5/1
  Selector26/1 -> Scope8/1
  Demux/1 -> Scope9/1
  Demux/2 -> Scope4/1
  Sum1/1 -> Scope12/1
  Selector28/1 -> Sum1/2, Scope14/1
  Selector27/1 -> Sum1/1
  Selector3/1 -> Solid Axle Suspension – Coil Spring/1, Selector27/1, Scope13/1
  Selector1/1 -> Solid Axle Suspension – Coil Spring/7, Selector28/1

== system CAVE_MachE_Testing_testing_V2/Vehicle Under Test1/Vehicle/Vehicle Dynamics/Vehicle 14DOF/Suspension/MacPherson Suspension ==
  Wheel : Inport
  Steering : Inport  Port=2
  Vehicle : Inport  Port=3
  Bus Creator1 : BusCreator  Inputs=5
  Bus Creator2 : BusCreator  Inputs=2
  Bus Creator3 : BusCreator  Inputs=2
  Bus Creator4 : BusCreator  Inputs=6
  Bus Selector : BusSelector  OutputSignals=z,Re,zdot,Fx,Fy,M
  Bus Selector1 : BusSelector  OutputSignals=P,V
  Selector1 : Selector  NumberOfDimensions=2  IndexOptions=Index vector (dialog),Select all  Indices=1,1  OutputSizes=1,1
  Selector2 : Selector  NumberOfDimensions=2  IndexOptions=Index vector (dialog),Select all  Indices=2,1  OutputSizes=1,1
  Steer Rate Adapter : Subsystem
  Steering Adapter : Subsystem
  Terminator : Terminator
  Vehicle Adapter : Subsystem
  Wheel  Adapter : Subsystem
  independent Suspensions - MacPherson : vehdynlibsuspension/Independent Suspension - MacPherson  ActiveDampEn=off  NumAxl=2  NumWhlsByAxl=[2 2]  StrgEnByAxl=[1 0]  AntiSwayEnByAxl=[1 0]  WhlNumVec="[1  2  1  2]"  AxleNumVec="[1  1  2  2]"  SuspTypesByAxle="[1  1]"  SuspImage=suspmacp.png  IdealSuspEn=on  IdealSuspAxles="[1  2]"  Kz=64370  F0z=9810  Cz=10000  Hmax=0.5  f_act_susp_cz=[10000 10000;10000 10000]  f_act_susp_duty_bpt=[0 1]  f_act_susp_zdot_bpt=[-1 1]  Toe=0.  RollStrgSlp=0.  ToeStrgSlp=0.  Caster=0.  CasterHslp=0.  CasterStrgSlp=0.  Camber=0.  CamberHslp=0.  CamberStrgSlp=0.  StrgHgtSlp=0.1432  MappedSuspEn=off  MappedSuspAxles="[1  2]"  f_susp_axl_bp=[1 2]  f_susp_dz_bp=[-0.15 -0.14 -0.13 -0.12 -0.11 -0.10 -0.09 -0.08 -0.07 -0.06 -0.05 -0.04 -0.03 -0.02 -0.01 0.00 0.01 0.02 0.03 0.04 0.05 0.06 0.07 0.08 0.09 0.10 0.11 0.12 0.13 0.14 0.15]  f_susp_dzdot_bp=[-0.15 -0.14 -0.13 -0.12 -0.11 -0.10 -0.09 -0.08 -0.07 -0.06 -0.05 -0.04 -0.03 -0.02 -0.01 0.00 0.01 0.02 0.03 0.04 0.05 0.06 0.07 0.08 0.09 0.10 0.11 0.12 0.13 0.14 0.15]  f_susp_fmz=zeros(31,31,61,2,4)  f_susp_geom=zeros(31,61,2,3)  f_susp_strgdelta_bp=[-30,-29,-28,-27,-26,-25,-24,-23,-22,-21,-20,-19,-18,-17,-16,-15,-14,-13,-12,-11,-10,-9,-8,-7,-6,-5,-4,-3,-2,-1,0,1,2,3,4,5,6,7,8,9,10,11,12,13,14,15,16,17,18,19,20,21,22,23,24,25,26,27,28,29,30]  AntiSwayR=0.2  AntiSwayNtrlAng=0.5236  AntiSwayTrsK=8e+02
  Suspension : Outport  VectorParamsAs1DForOutWhenUnconnected=off
  wires:
  independent Suspensions - MacPherson/1 -> Terminator/1  "Susp"
  Steering Adapter/1(StrgAng) -> independent Suspensions - MacPherson/9
  Steer Rate Adapter/1(AngVel) -> Bus Creator1/5  "AngVel"
  Bus Creator4/1 -> Bus Selector/1
  Bus Creator2/1 -> Bus Creator3/1  "Veh"
  independent Suspensions - MacPherson/2 -> Bus Creator2/1  "F"
  independent Suspensions - MacPherson/5 -> Selector1/1, Selector2/1  "V"
  independent Suspensions - MacPherson/6 -> Bus Creator1/4  "Ang"
  independent Suspensions - MacPherson/4 -> Bus Creator1/1  "F"
  Bus Selector/1 -> independent Suspensions - MacPherson/1  "<z>"
  Bus Selector1/1 -> independent Suspensions - MacPherson/7  "<P>"
  Selector2/1 -> Bus Creator1/3  "ydot"
  Selector1/1 -> Bus Creator1/2  "xdot"
  Bus Selector/2 -> independent Suspensions - MacPherson/2  "<Re>"
  Wheel  Adapter/6(Re) -> Bus Creator4/6
  Wheel  Adapter/5(M) -> Bus Creator4/5  "M"
  Wheel  Adapter/4(zdot) -> Bus Creator4/4
  Wheel  Adapter/3(z) -> Bus Creator4/3
  Wheel/1 -> Wheel  Adapter/1(Wheels)
  Wheel  Adapter/1(WhlFx) -> Bus Creator4/1  "Fx"
  Wheel  Adapter/2(WhlFy) -> Bus Creator4/2  "Fy"
  independent Suspensions - MacPherson/3 -> Bus Creator2/2  "M"
  Vehicle Adapter/1(VehSusp) -> Bus Selector1/1
  Vehicle/1 -> Vehicle Adapter/1(Veh), Steer Rate Adapter/1(Veh)
  Bus Selector/4 -> independent Suspensions - MacPherson/4  "<Fx>"
  Bus Selector/3 -> independent Suspensions - MacPherson/3  "<zdot>"
  Steering/1 -> Steering Adapter/1(Steer)
  Bus Selector/5 -> independent Suspensions - MacPherson/5  "<Fy>"
  Bus Selector/6 -> independent Suspensions - MacPherson/6  "<M>"
  Bus Selector1/2 -> independent Suspensions - MacPherson/8  "<V>"
  Bus Creator1/1 -> Bus Creator3/2  "Whl"
  Bus Creator3/1 -> Suspension/1

== system CAVE_MachE_Testing_testing_V2/Vehicle Under Test1/Vehicle/Vehicle Dynamics/Vehicle 14DOF/Suspension/Mapped Suspension ==
  Wheel : Inport
  Steering : Inport  Port=2
  Vehicle : Inport  Port=3
  Bus Creator1 : BusCreator  Inputs=5
  Bus Creator2 : BusCreator  Inputs=2
  Bus Creator3 : BusCreator  Inputs=2
  Bus Creator4 : BusCreator  Inputs=6
  Bus Selector : BusSelector  OutputSignals=z,Re,zdot,Fx,Fy,M
  Bus Selector1 : BusSelector  OutputSignals=P,V
  Independent Suspension - Mapped : vehdynlibsuspension/Independent Suspension - Mapped  NumAxl=2  NumWhlsByAxl=[2 2]  StrgEnByAxl=[1 0]  AntiSwayEnByAxl=[1 0]  WhlNumVec="[1  2  1  2]"  AxleNumVec="[1  1  2  2]"  SuspTypesByAxle="[2  2]"  SuspImage=suspindmap.png  IdealSuspEn=off  IdealSuspAxles="[1  2]"  Kz=64370  F0z=9810  Cz=10000  Hmax=0.5  Toe=2  RollStrgSlp=-13  ToeStrgSlp=0.01  Caster=4  CasterHslp=-13  CasterStrgSlp=0.01  Camber=4  CamberHslp=-13  CamberStrgSlp=0.01  StrgHgtSlp=0.0025  MappedSuspEn=on  MappedSuspAxles="[1  2]"  f_susp_axl_bp=[1 2]  f_susp_dz_bp=f_susp_dz_bp  f_susp_dzdot_bp=f_susp_dzdot_bp  f_susp_fmz=f_susp_fmz  f_susp_geom=f_susp_geom  f_susp_strgdelta_bp=f_susp_strgdelta_bp  NDFLookupOutType=1:4  NDGLookupOutType=1:3  AntiSwayR=0.2  AntiSwayNtrlAng=0.5236  AntiSwayTrsK=8e2
      link override For each track and axle combination calculate suspension forces and moments/Suspension/Suspension Angle Calculations: OverrideUsingVariant=MappedSteeringEnabled
      link override For each track and axle combination calculate suspension forces and moments/Suspension/Z axis suspension characteristic: OverrideUsingVariant=MappedSuspension
  Reshape1 : Reshape  OutputDimensionality=Row vector (2-D)
  Selector : Selector  IndexOptions=Index vector (dialog)  Indices=[1 2]  OutputSizes=1
  Selector1 : Selector  NumberOfDimensions=2  IndexOptions=Index vector (dialog),Select all  Indices=1,1  OutputSizes=1,1
  Selector2 : Selector  NumberOfDimensions=2  IndexOptions=Index vector (dialog),Select all  Indices=2,1  OutputSizes=1,1
  Steer Rate Adapter : Subsystem
  Terminator : Terminator
  Vehicle Adapter : Subsystem
  Wheel  Adapter : Subsystem
  Suspension : Outport  VectorParamsAs1DForOutWhenUnconnected=off
  wires:
  Steer Rate Adapter/1(AngVel) -> Bus Creator1/5
  Bus Creator3/1 -> Suspension/1
  Independent Suspension - Mapped/5 -> Selector1/1, Selector2/1  "V"
  Selector1/1 -> Bus Creator1/2  "xdot"
  Independent Suspension - Mapped/4 -> Bus Creator1/1  "F"
  Bus Creator1/1 -> Bus Creator3/2  "Whl"
  Bus Creator2/1 -> Bus Creator3/1  "Veh"
  Independent Suspension - Mapped/3 -> Bus Creator2/2  "M"
  Independent Suspension - Mapped/2 -> Bus Creator2/1  "F"
  Selector2/1 -> Bus Creator1/3  "ydot"
  Independent Suspension - Mapped/6 -> Bus Creator1/4  "Ang"
  Vehicle/1 -> Vehicle Adapter/1(Veh), Steer Rate Adapter/1(Veh)
  Steering/1 -> Selector/1
  Bus Selector1/1 -> Independent Suspension - Mapped/7  "<P>"
  Wheel  Adapter/1(WhlFx) -> Bus Creator4/1  "Fx"
  Bus Selector/1 -> Independent Suspension - Mapped/1  "<z>"
  Bus Selector/3 -> Independent Suspension - Mapped/3  "<zdot>"
  Vehicle Adapter/1(VehSusp) -> Bus Selector1/1
  Wheel/1 -> Wheel  Adapter/1(Wheels)
  Wheel  Adapter/2(WhlFy) -> Bus Creator4/2  "Fy"
  Wheel  Adapter/3(z) -> Bus Creator4/3
  Bus Creator4/1 -> Bus Selector/1
  Selector/1 -> Reshape1/1
  Wheel  Adapter/6(Re) -> Bus Creator4/6
  Wheel  Adapter/4(zdot) -> Bus Creator4/4
  Bus Selector/6 -> Independent Suspension - Mapped/6  "<M>"
  Wheel  Adapter/5(M) -> Bus Creator4/5
  Bus Selector/4 -> Independent Suspension - Mapped/4  "<Fx>"
  Bus Selector1/2 -> Independent Suspension - Mapped/8  "<V>"
  Bus Selector/2 -> Independent Suspension - Mapped/2  "<Re>"
  Bus Selector/5 -> Independent Suspension - Mapped/5  "<Fy>"
  Reshape1/1 -> Independent Suspension - Mapped/9
  Independent Suspension - Mapped/1 -> Terminator/1  "Susp"

== system CAVE_MachE_Testing_testing_V2/Vehicle Under Test1/Vehicle/Vehicle Dynamics/Vehicle 14DOF/Vehicle/Variant Subsystem ==
  note: 1) Add Subsystem or Model blocks as valid variant choices.
      | 2) You cannot connect blocks at this level. At simulation, connectivity is automatically
      | determined, based on the active variant and port name matching.
  Suspension : Inport
  Wind : Inport  Port=2
  3DOF : Subsystem  VariantControl=0
  6DOF : Subsystem  VariantControl=1
  VehFdbk : Outport  VectorParamsAs1DForOutWhenUnconnected=off

== system CAVE_MachE_Testing_testing_V2/Vehicle Under Test1/Vehicle/Vehicle Dynamics/Vehicle 14DOF/Wheels and Tires/VDBS ==
  WheelAng : Inport
  CamberAng : Inport  Port=2  Unit=rad
  AxleTrq : Inport  Port=3
  BrkPrs : Inport  Port=4
  Fz : Inport  Port=5  Unit=N
  r : Inport  Port=6
  VehVel : Inport  Port=7
  Ground Level : Inport  Port=8
  Friction : Inport  Port=9  Unit=1  PortDimensions=4
  Bus Selector : BusSelector  OutputSignals=z
  Pressure : vehdynlibtirecommon/Constant  const=220000  numWheels=4
  Scope{,1..4} (5 alike) : Scope
  Terminator : Terminator
  Tire2Veh : Subsystem
  Tires : Subsystem  Variant=on  VariantControlMode=label  VariantControl=Variant1  LabelModeActiveChoice=0
  Veh2Tire : Subsystem
  scale factors with friction : Subsystem  mask{numWheels=4}
      mask prompts: numWheels "Number of wheels"
  Wheels : Outport  VectorParamsAs1DForOutWhenUnconnected=off
  FrntAxlF : Outport  Port=2  Unit=N  VectorParamsAs1DForOutWhenUnconnected=off
  RearAxlF : Outport  Port=3  Unit=N  VectorParamsAs1DForOutWhenUnconnected=off
  Omega : Outport  Port=4  VectorParamsAs1DForOutWhenUnconnected=off
  Mz : Outport  Port=5  Unit=N*m  VectorParamsAs1DForOutWhenUnconnected=off
  SuspWhlPz : Outport  Port=6  VectorParamsAs1DForOutWhenUnconnected=off
  SuspWhlVz : Outport  Port=7  VectorParamsAs1DForOutWhenUnconnected=off
  wires:
  Tire2Veh/1(Wheels) -> Wheels/1
  CamberAng/1 -> Veh2Tire/6(WheelCamber), Tire2Veh/3(WheelCamber), Tires/6("Camber ")
  Tire2Veh/7(SuspWhlVz) -> SuspWhlVz/1
  Tire2Veh/6(SuspWhlPz) -> SuspWhlPz/1
  Veh2Tire/6(zdotAxle) -> Terminator/1
  r/1 -> Veh2Tire/1(r)
  Friction/1 -> scale factors with friction/2(lamda_mu_y), scale factors with friction/1(lamda_mu_x)
  Tire2Veh/5(<Mz>) -> Mz/1
  Tire2Veh/4(RearAxlF) -> RearAxlF/1
  Tire2Veh/3(FrntAxlF) -> FrntAxlF/1
  Tire2Veh/2(Omega) -> Omega/1, Scope/1
  WheelAng/1 -> Tire2Veh/4(WheelSteer), Veh2Tire/5(WheelSteer)
  Tires/1(" Wheels") -> Bus Selector/1, Tire2Veh/1(Wheel)
  Veh2Tire/3(psidot) -> Tires/3("r ")
  Veh2Tire/5(ydotAxle) -> Tires/5("Vy ")
  Veh2Tire/4(xdotAxle) -> Tires/4("Vx ")
  Veh2Tire/2(P) -> Tires/2("Brake Pressure ")
  Veh2Tire/1(T) -> Scope1/1, Tires/1("DriveTorque ")
  VehVel/1 -> Veh2Tire/4(VehVel)
  BrkPrs/1 -> Veh2Tire/3(Brake)
  AxleTrq/1 -> Scope2/1, Veh2Tire/2(Axle)
  Fz/1 -> Tire2Veh/2(Fz), Tires/10("FzSusp ")
  scale factors with friction/1(lambdas) -> Tires/8("lambda ")
  Pressure/1 -> Tires/7("Press ")
  Ground Level/1 -> Scope3/1, Tires/9("Gnd ")
  Bus Selector/1 -> Scope4/1  "<z>"

== system CAVE_MachE_Testing_testing_V2/Vehicle Under Test1/Vehicle/Vehicle Dynamics/Vehicle 7DOF/Longitudinal Wheels 4DOF/Axle Forces ==
  note: 1) Add Subsystem or Model blocks as valid variant choices.
      | 2) You cannot connect blocks at this level. At simulation, connectivity is automatically
      | determined, based on the active variant and port name matching.
  F : Inport
  R : Inport  Port=2
  Bicycle : Subsystem  VariantControl=0
  Dual : Subsystem  VariantControl=1
  FrntAxlF : Outport  Unit=N  VectorParamsAs1DForOutWhenUnconnected=off
  RearAxlF : Outport  Port=2  Unit=N  VectorParamsAs1DForOutWhenUnconnected=off
